simulink model "Acquisition_mine"  (R2019b)
settings: Solver=VariableStepAuto  StartTime=0.0  StopTime=0.0081  FixedStep=1/fs  RelTol=1e-3  EnableMultiTasking=on
values from neighbouring files (symbols this model uses):
  freq_vector = 2*pi*[(fc - 10e3):1e3:(fc+10e3)]    [config.m]
  fs = 16367600    [config.m]
  fs_fft = 2^15*1e3    (= 32768000)    [config.m]
  Len = ceil(ms*fs/1000)    [config.m]
  Len_fft = fs_fft*ms/1000    (= 32768)    [config.m]
undefined symbols (not defined in the file or in its folder): __PRM__SERIALIZED__DATA__, SubsystemReferenceBlock
libraries: commseqgen3 x4, dspsigops x4, dspstat3 x3, dspsrcs4 x2, simulink x1
settings Model: Creator=nishantmittal  LastModifiedBy=nishantmittal
settings SolverCC: AutoInsertRateTranBlk=on
settings OptimizationCC: DefaultUnderspecifiedDataType=single
settings DebuggingCC: ParameterPrecisionLossMsg=none

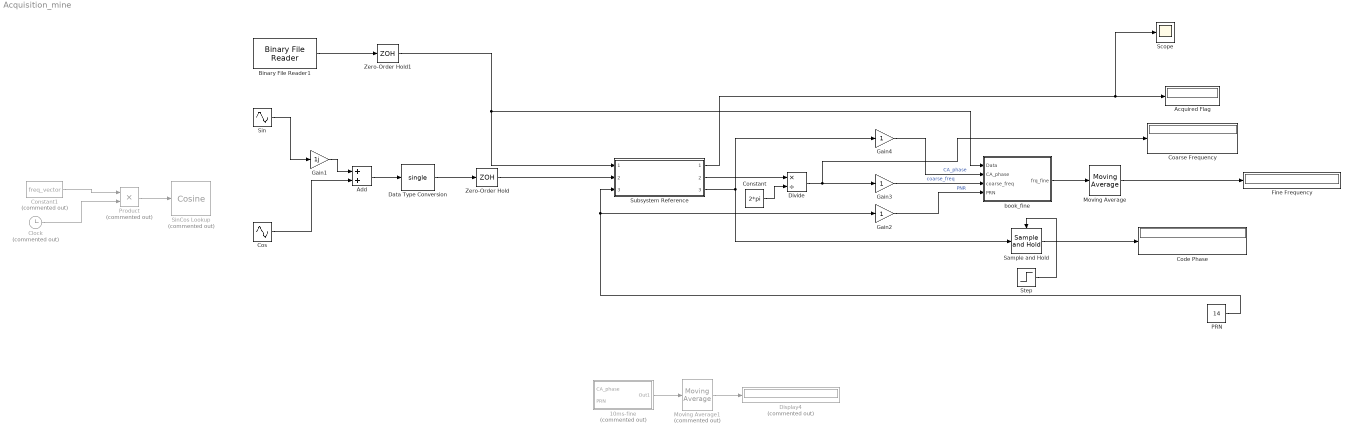
== system Acquisition_mine ==
  10ms-fine : Subsystem  Commented=on
  Acquired Flag : Display
  Add : Sum
  Binary File Reader1 : dspsrcs4/Binary File Reader  Filename=/Users/nishantmittal/Documents/SURP/data/Acqisition/test/gioveAandB_short.bin  HeaderStructure=struct([])  DataType=int8  SamplesPerFrame=1  IsDataComplex=off  NumChannels=1  OutputEOF=off  SampleTime=1/fs  SimulateUsing=Code generation
      settings: SourceProductName=DSP System Toolbox  SourceProductBaseCode=DS
  Clock : Clock  Commented=on
  Coarse Frequency : Display
  Code Phase : Display
  Constant : Constant  Value=2*pi  OutDataTypeStr=single
  Constant1 : Constant  Commented=on  Value=freq_vector
  Cos : Sin  Frequency=freq_vector  Phase=pi/2  SampleTime=1/fs
  Data Type Conversion : DataTypeConversion  OutDataTypeStr=single
  Display4 : Display  Commented=on
  Divide : Product  Inputs=*/
  Fine Frequency : Display
  Gain1 : Gain  Gain=1j
  Gain2 : Gain
  Gain3 : Gain
  Gain4 : Gain  OutDataTypeStr=single
  Moving Average : dspstat3/Moving Average  Method=Sliding window  ForgettingFactorPort=off  SpecifyWindowLength=on  WindowLength=4  ForgettingFactor=0.9  SimulateUsing=Code generation
  Moving Average1 : dspstat3/Moving Average  Commented=on  Method=Sliding window  ForgettingFactorPort=off  SpecifyWindowLength=on  WindowLength=2  ForgettingFactor=0.9  SimulateUsing=Code generation
  "PRN " : Constant  Value=14  OutDataTypeStr=single
  Product : Product  Commented=on
  Sample and Hold : dspsigops/Sample and Hold  trig=Rising edge  initCond=0  latchinput=off
  Scope : Scope
  "Sin " : Sin  Frequency=freq_vector  SampleTime=1/fs
  SinCos Lookup : simulink/Lookup Tables/Cosine  Commented=on  Formula=sin(2*pi*u) and cos(2*pi*u)  NumDataPoints=(2^14)+1  OutputWordLength=16  InternalRulePriority=Speed
      settings: SourceProductName=Simulink  SourceProductBaseCode=SL
  Step : Step  Time=0.00101  SampleTime=0
  Subsystem Reference : Subsystem  BlockKeywords=__PRM__SERIALIZED__DATA__:SubsystemReferenceBlock  ReferencedSubsystem=acq_PNR
      settings: MinAlgLoopOccurrences=on
  Zero-Order Hold : ZeroOrderHold  SampleTime=1/fs_fft
  Zero-Order Hold1 : ZeroOrderHold  SampleTime=1/fs_fft
  book_fine : Subsystem
  wires:
  Gain1/1 -> Add/1
  Add/1 -> Data Type Conversion/1
  "PRN "/1 -> Subsystem Reference/3, Gain2/1
  Subsystem Reference/3 -> Sample and Hold/1, Gain4/1
  Subsystem Reference/1 -> Scope/1, Acquired Flag/1
  Divide/1 -> Gain3/1, Coarse Frequency/1
  Subsystem Reference/2 -> Divide/1
  Constant/1 -> Divide/2
  Gain4/1 -> book_fine/2(CA_phase)  "CA_phase"
  10ms-fine/1(Out1) -> Moving Average1/1
  Gain2/1 -> book_fine/4(PRN)  "PNR"
  Gain3/1 -> book_fine/3(coarse_freq)  "coarse_freq"
  Moving Average1/1 -> Display4/1
  Step/1 -> Sample and Hold/Trigger
  book_fine/1(frq_fine) -> Moving Average/1
  Moving Average/1 -> Fine Frequency/1
  Sample and Hold/1 -> Code Phase/1
  Product/1 -> SinCos Lookup/1
  Clock/1 -> Product/2
  Constant1/1 -> Product/1
  Zero-Order Hold/1 -> Subsystem Reference/2
  Data Type Conversion/1 -> Zero-Order Hold/1
  Cos/1 -> Add/2
  "Sin "/1 -> Gain1/1
  Binary File Reader1/1 -> Zero-Order Hold1/1
  Zero-Order Hold1/1 -> book_fine/1(Data), Subsystem Reference/1

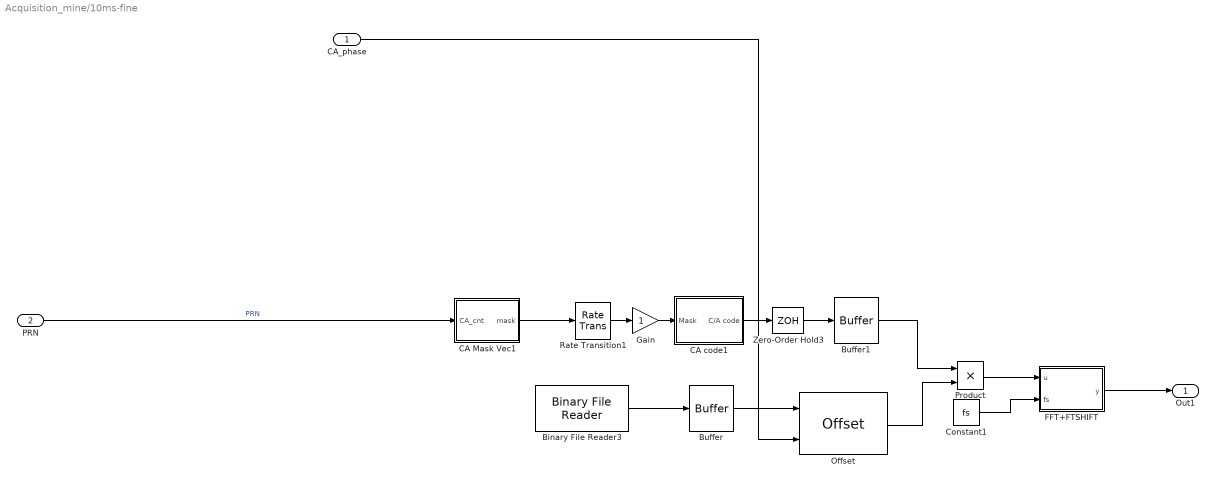
== system Acquisition_mine/10ms-fine ==
  CA_phase : Inport
  PRN : Inport  Port=2
  Binary File Reader3 : dspsrcs4/Binary File Reader  Filename=/Users/nishantmittal/Documents/SURP/data/Acqisition/test/gioveAandB_short.bin  HeaderStructure=struct([])  DataType=int8  SamplesPerFrame=1  IsDataComplex=off  NumChannels=1  OutputEOF=off  SampleTime=1/fs  SimulateUsing=Code generation
      settings: SourceProductName=DSP System Toolbox  SourceProductBaseCode=DS
  Buffer : Buffer  N=11*Len  OutputFrames=off
  Buffer1 : Buffer  N=10*Len  OutputFrames=off
  CA Mask Vec1 : MATLAB Function  TreatAsAtomicUnit=on
  CA code1 : Subsystem
  Constant1 : Constant  Value=fs
  FFT+FTSHIFT : MATLAB Function  TreatAsAtomicUnit=on
  Gain : Gain
  Offset : dspsigops/Offset  mode=Remove beginning samples  numDatOffPair=1  outWidthSpec=User-defined  outWidth=10*Len  actionOutRange=Clip
      settings: SourceProductName=DSP System Toolbox  SourceProductBaseCode=DS
  Product : Product
  Rate Transition1 : RateTransition  Deterministic=off  OutPortSampleTime=1/(1.023e6)
  Zero-Order Hold3 : ZeroOrderHold  SampleTime=1/fs
  Out1 : Outport
  wires:
  CA_phase/1 -> Offset/2
  Rate Transition1/1 -> Gain/1
  Binary File Reader3/1 -> Buffer/1
  Constant1/1 -> FFT+FTSHIFT/2(fs)
  CA Mask Vec1/1(mask) -> Rate Transition1/1
  Buffer1/1 -> Product/1
  FFT+FTSHIFT/1(y) -> Out1/1
  Gain/1 -> CA code1/1(Mask)
  Zero-Order Hold3/1 -> Buffer1/1
  PRN/1 -> CA Mask Vec1/1(CA_cnt)  "PRN"
  Buffer/1 -> Offset/1
  Product/1 -> FFT+FTSHIFT/1(u)
  Offset/1 -> Product/2
  CA code1/1(C/A code) -> Zero-Order Hold3/1

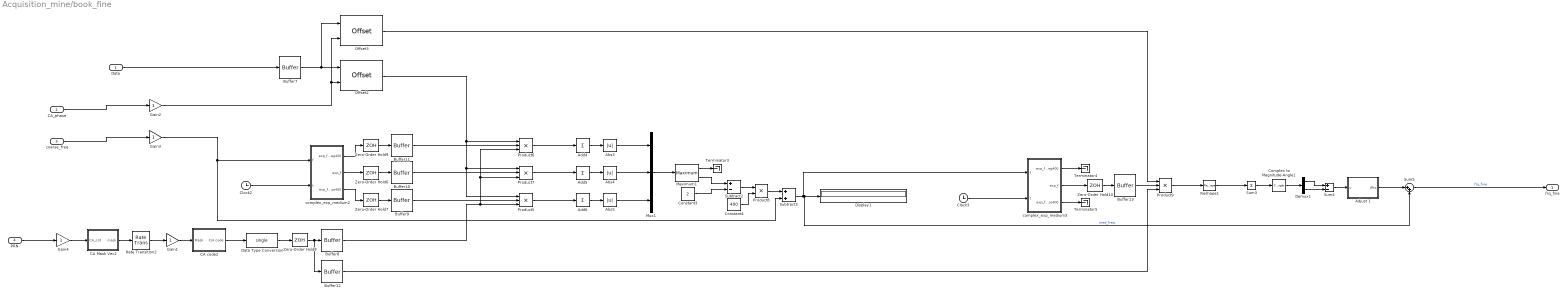
== system Acquisition_mine/book_fine ==
  Data : Inport
  CA_phase : Inport  Port=2
  coarse_freq : Inport  Port=3
  PRN : Inport  Port=4
  Abs3 : Abs
  Abs4 : Abs
  Abs5 : Abs
  Add4 : Sum  Inputs=+
  Add5 : Sum  Inputs=+
  Add6 : Sum  Inputs=+
  Adjust 1 : MATLAB Function  TreatAsAtomicUnit=on
  Buffer{8..11} (4 alike) : Buffer  N=Len_fft  OutputFrames=off
  Buffer12 : Buffer  N=2*Len_fft  OutputFrames=off
  Buffer13 : Buffer  N=2*Len_fft  OutputFrames=off
  Buffer7 : Buffer  N=3*Len_fft  OutputFrames=off
  CA Mask Vec2 : MATLAB Function  TreatAsAtomicUnit=on
  CA code2 : Subsystem
  Clock2 : Clock
  Clock3 : Clock
  Complex to Magnitude-Angle1 : ComplexToMagnitudeAngle  Output=Angle
  Constant3 : Constant  Value=2  OutDataTypeStr=single
  Constant4 : Constant  Value=400  OutDataTypeStr=single
  Data Type Conversion : DataTypeConversion  OutDataTypeStr=single
  Demux1 : Demux  Outputs=2
  Display1 : Display
  Gain1 : Gain  OutDataTypeStr=uint8
  Gain2 : Gain
  Gain3 : Gain
  Gain4 : Gain
  Maximum1 : dspstat3/Maximum  operation=maximum  fcn=Value and Index  indexBase=One  operateOver=Each column  Dimension=1  InputProcessing=Columns as channels (frame based)  reset=None  roiEnable=off  roiType=Rectangles  roiPortion=Entire ROI  roiOutput=Individual statistics for each ROI  roiFlag=off  roundingMode=Floor  overflowMode=off  accumDataTypeStr=Inherit: Same as product output  accumLastDataTypeStr=Inherit: Same as product output
  Mux1 : Mux  Inputs=3
  Offset2 : dspsigops/Offset  mode=Remove beginning samples  numDatOffPair=1  outWidthSpec=User-defined  outWidth=Len_fft  actionOutRange=Clip
      settings: SourceProductName=DSP System Toolbox  SourceProductBaseCode=DS
  Offset3 : dspsigops/Offset  mode=Remove beginning samples  numDatOffPair=1  outWidthSpec=User-defined  outWidth=2*Len_fft  actionOutRange=Clip
      settings: SourceProductName=DSP System Toolbox  SourceProductBaseCode=DS
  Product{5..7,9} (4 alike) : Product  Inputs=3
  Product8 : Product
  Rate Transition2 : RateTransition  Deterministic=off  OutPortSampleTime=1/(1.023e6)
  Reshape1 : Reshape  OutputDimensionality=Customize  OutputDimensions=[Len_fft,2]
  Subtract2 : Sum  Inputs=+-
  Subtract3 : Sum
  Sum3 : Sum  Inputs=+  CollapseMode=Specified dimension
  Sum4 : Sum  Inputs=+-
  Sum5 : Sum  Inputs=|++
  Terminator3 : Terminator
  Terminator4 : Terminator
  Terminator5 : Terminator
  Zero-Order Hold{6..10} (5 alike) : ZeroOrderHold  SampleTime=1/fs_fft
  complex_exp_medium2 : MATLAB Function  TreatAsAtomicUnit=on
  complex_exp_medium3 : MATLAB Function  TreatAsAtomicUnit=on
  frq_fine : Outport
  wires:
  Complex to Magnitude-Angle1/1 -> Demux1/1
  Add6/1 -> Abs5/1
  Clock2/1 -> complex_exp_medium2/2(t)
  Subtract3/1 -> complex_exp_medium3/1(f), Sum5/2, Display1/1  "med_freq"
  Product9/1 -> Reshape1/1
  Demux1/1 -> Sum4/1
  Constant3/1 -> Subtract2/2
  Buffer11/1 -> Product6/2
  Buffer13/1 -> Product9/2
  Abs5/1 -> Mux1/3
  Gain1/1 -> CA code2/1(Mask)
  Add4/1 -> Abs3/1
  Sum3/1 -> Complex to Magnitude-Angle1/1
  Clock3/1 -> complex_exp_medium3/2(t)
  Maximum1/1 -> Terminator3/1
  Constant4/1 -> Product8/2
  Demux1/2 -> Sum4/2
  Buffer8/1 -> Product6/3, Product7/3, Product5/3
  Offset3/1 -> Product9/1
  Buffer7/1 -> Offset3/1, Offset2/1
  complex_exp_medium3/2(exp_f) -> Zero-Order Hold10/1
  Add5/1 -> Abs4/1
  Product5/1 -> Add6/1
  Mux1/1 -> Maximum1/1
  Zero-Order Hold8/1 -> Buffer12/1, Buffer8/1
  Adjust 1/1(dfrq) -> Sum5/1
  Reshape1/1 -> Sum3/1
  complex_exp_medium2/2(exp_f) -> Zero-Order Hold6/1
  Buffer10/1 -> Product7/2
  Product8/1 -> Subtract3/1
  Buffer12/1 -> Product9/3
  Rate Transition2/1 -> Gain1/1
  Abs4/1 -> Mux1/2
  Buffer9/1 -> Product5/2
  Subtract2/1 -> Product8/1
  Zero-Order Hold9/1 -> Buffer11/1
  Product7/1 -> Add5/1
  complex_exp_medium2/3(exp_f_pos400) -> Zero-Order Hold7/1
  Sum4/1 -> Adjust 1/1(u)
  CA code2/1(C/A code) -> Data Type Conversion/1
  Zero-Order Hold7/1 -> Buffer9/1
  Product6/1 -> Add4/1
  Zero-Order Hold6/1 -> Buffer10/1
  CA Mask Vec2/1(mask) -> Rate Transition2/1
  Abs3/1 -> Mux1/1
  complex_exp_medium2/1(exp_f_neg400) -> Zero-Order Hold9/1
  complex_exp_medium3/3(exp_f_pos400) -> Terminator5/1
  Sum5/1 -> frq_fine/1  "frq_fine"
  complex_exp_medium3/1(exp_f_neg400) -> Terminator4/1
  Zero-Order Hold10/1 -> Buffer13/1
  Offset2/1 -> Product5/1, Product7/1, Product6/1
  Maximum1/2 -> Subtract2/1
  Gain2/1 -> Offset3/2, Offset2/2
  Gain3/1 -> Subtract3/2, complex_exp_medium2/1(f)
  Gain4/1 -> CA Mask Vec2/1(CA_cnt)
  PRN/1 -> Gain4/1
  coarse_freq/1 -> Gain3/1
  CA_phase/1 -> Gain2/1
  Data/1 -> Buffer7/1
  Data Type Conversion/1 -> Zero-Order Hold8/1

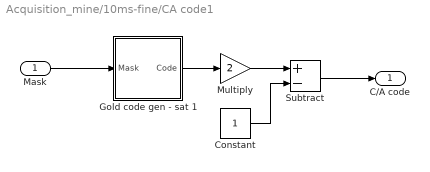
== system Acquisition_mine/10ms-fine/CA code1 ==
  Mask : Inport
  Constant : Constant
  Gold code gen - sat 1 : Subsystem
  Multiply : Gain  Gain=2
  Subtract : Sum  Inputs=+-
  C/A code : Outport
  wires:
  Subtract/1 -> C/A code/1
  Multiply/1 -> Subtract/1
  Gold code gen - sat 1/1(Code) -> Multiply/1
  Constant/1 -> Subtract/2
  Mask/1 -> Gold code gen - sat 1/1(Mask)

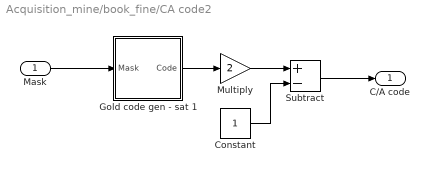
== system Acquisition_mine/book_fine/CA code2 ==
  Mask : Inport
  Constant : Constant
  Gold code gen - sat 1 : Subsystem
  Multiply : Gain  Gain=2
  Subtract : Sum  Inputs=+-
  C/A code : Outport
  wires:
  Subtract/1 -> C/A code/1
  Multiply/1 -> Subtract/1
  Gold code gen - sat 1/1(Code) -> Multiply/1
  Constant/1 -> Subtract/2
  Mask/1 -> Gold code gen - sat 1/1(Mask)

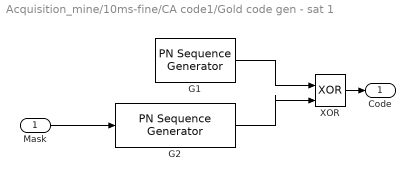
== system Acquisition_mine/10ms-fine/CA code1/Gold code gen - sat 1 ==
  Mask : Inport
  G1 : commseqgen3/PN Sequence Generator  poly=[10 7 0]  ini_sta=[1 1 1 1 1 1 1 1 1 1]  outBitMaskSource=Dialog parameter  shift=[0 0 0 0 0 0 0 0 0 1]  outVarSiz=off  maxOutSizeMode=Dialog parameter  maxOutSize=[10 1]  Ts=1/(1.023e6)  sampPerFrame=1  reset=off  bitPackedOutputs=off  outDataType=boolean  numPackedBits=8  bitPackDataSigned=off  bitPackedOutDType=double
      settings: SourceProductName=Communications Toolbox
  G2 : commseqgen3/PN Sequence Generator  poly=[10 8 7 4 2 1 0]  ini_sta=[1 1 1 1 1 1 1 1 1 1]  outBitMaskSource=Input port  shift=[0 1 0 0 0 1 0 0 0 0]  outVarSiz=off  maxOutSizeMode=Dialog parameter  maxOutSize=[10 1]  Ts=1/(1.023e6)  sampPerFrame=1  reset=off  bitPackedOutputs=off  outDataType=boolean  numPackedBits=8  bitPackDataSigned=off  bitPackedOutDType=double
      settings: SourceProductName=Communications Toolbox
  XOR : Logic  Operator=XOR  IconShape=distinctive  AllPortsSameDT=off  OutDataTypeStr=boolean
  Code : Outport
  wires:
  G2/1 -> XOR/2
  XOR/1 -> Code/1
  G1/1 -> XOR/1
  Mask/1 -> G2/1

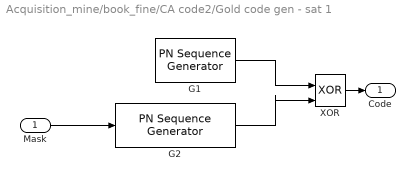
== system Acquisition_mine/book_fine/CA code2/Gold code gen - sat 1 ==
  Mask : Inport
  G1 : commseqgen3/PN Sequence Generator  poly=[10 7 0]  ini_sta=[1 1 1 1 1 1 1 1 1 1]  outBitMaskSource=Dialog parameter  shift=[0 0 0 0 0 0 0 0 0 1]  outVarSiz=off  maxOutSizeMode=Dialog parameter  maxOutSize=[10 1]  Ts=1/(1.023e6)  sampPerFrame=1  reset=off  bitPackedOutputs=off  outDataType=boolean  numPackedBits=8  bitPackDataSigned=off  bitPackedOutDType=double
      settings: SourceProductName=Communications Toolbox
  G2 : commseqgen3/PN Sequence Generator  poly=[10 8 7 4 2 1 0]  ini_sta=[1 1 1 1 1 1 1 1 1 1]  outBitMaskSource=Input port  shift=[0 1 0 0 0 1 0 0 0 0]  outVarSiz=off  maxOutSizeMode=Dialog parameter  maxOutSize=[10 1]  Ts=1/(1.023e6)  sampPerFrame=1  reset=off  bitPackedOutputs=off  outDataType=boolean  numPackedBits=8  bitPackDataSigned=off  bitPackedOutDType=double
      settings: SourceProductName=Communications Toolbox
  XOR : Logic  Operator=XOR  IconShape=distinctive  AllPortsSameDT=off  OutDataTypeStr=boolean
  Code : Outport
  wires:
  G2/1 -> XOR/2
  XOR/1 -> Code/1
  G1/1 -> XOR/1
  Mask/1 -> G2/1

== matlab function Acquisition_mine/10ms-fine/CA Mask Vec1 ==
  data: CA_cnt input; mask output
function mask = fcn(CA_cnt)

phase = [2 6; 3 7; 4 8; 5 9; 1 9; 2 10; 1 8; 2 9; 3 10; 2 3; 3 4; 5 6; 6 7; 7 8; 8 9; 9 10; 1 4; 2 5; 3 6; 4 7; 5 8; 6 9; 1 3; 4 6; 5 7; 6 8; 7 9; 8 10; 1 6; 2 7; 3 8; 4 9];
mask_points = phase(CA_cnt, :);
mask = zeros(1,10);
mask(mask_points) = 1;

== matlab function Acquisition_mine/10ms-fine/FFT+FTSHIFT ==
  data: u input; y output; fs input
function y = fcn(u, fs)
temp = fftshift(fft(u));
l = length(temp);
temp2 = temp(l/2+1:end);
[~, index] = max(temp2);
y = (index-1)*fs/l;

== matlab function Acquisition_mine/book_fine/Adjust 1 ==
  data: u input; dfrq output
function dfrq = fcn(u)
u = u/(2*pi);
temp = u;
threshold = 0.23; 
if abs(u)>threshold% for angle adjustment 
    u = temp-1;
    if abs(u)>threshold
        u = temp+1; % end
        if abs(u)>0.22 % for pi phase shift correction
            u = temp-0.5;
            if abs(u)>threshold
                u = temp - 1.5;
                if abs(u)>threshold
                    u = temp+0.5;
                end
            end
        end
    end
end
dfrq = u*1000;

== matlab function Acquisition_mine/book_fine/CA Mask Vec2 ==
  data: CA_cnt input; mask output
function mask = fcn(CA_cnt)

phase = [2 6; 3 7; 4 8; 5 9; 1 9; 2 10; 1 8; 2 9; 3 10; 2 3; 3 4; 5 6; 6 7; 7 8; 8 9; 9 10; 1 4; 2 5; 3 6; 4 7; 5 8; 6 9; 1 3; 4 6; 5 7; 6 8; 7 9; 8 10; 1 6; 2 7; 3 8; 4 9];
mask_points = phase(CA_cnt, :);
mask = zeros(1,10);
mask(mask_points) = 1;

== matlab function Acquisition_mine/book_fine/complex_exp_medium2 ==
  data: exp_f_neg400 output; f input; exp_f output; t input; exp_f_pos400 output
function [exp_f_neg400, exp_f, exp_f_pos400] = fcn(f, t)
exp_f_neg400 = exp(1i*2*pi*(f-400)*t);
exp_f = exp(1i*2*pi*f*t);
exp_f_pos400 = exp(1i*2*pi*(f+400)*t);

== matlab function Acquisition_mine/book_fine/complex_exp_medium3 ==
  data: exp_f_neg400 output; f input; exp_f output; t input; exp_f_pos400 output
function [exp_f_neg400, exp_f, exp_f_pos400] = fcn(f, t)
exp_f_neg400 = exp(1i*2*pi*(f-400)*t);
exp_f = exp(1i*2*pi*f*t);
exp_f_pos400 = exp(1i*2*pi*(f+400)*t);
